simulink model "Robot_diferencial_trayectoria_senoidal"  (R2017b)
settings: Solver=VariableStepAuto  StartTime=0.0  StopTime=Tsim  MaxStep=1e-2  MinStep=1e-7  RelTol=1e-3
values from neighbouring files (symbols this model uses):
  A = 0.25    [graf.m]
  accel_limit = 15    [graf.m]
  B = 1    [graf.m]
  CI = [0 0 0]    [graf.m]
libraries: simulink_need_slupdate x1
settings Model: Creator=Raúl  LastModifiedBy=Alvaro

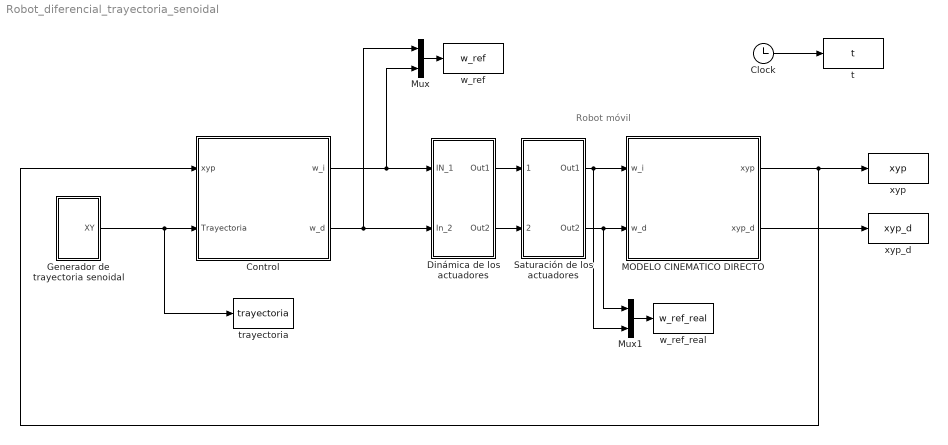
== system Robot_diferencial_trayectoria_senoidal ==
  note: Robot móvil
  Clock : Clock
  "Control " : Subsystem
  Dinámica de los actuadores : Subsystem
  Generador de trayectoria senoidal : Subsystem
  MODELO CINEMATICO DIRECTO : Subsystem
  Mux : Mux  Inputs=2
  Mux1 : Mux  Inputs=2
  Saturación de los actuadores : Subsystem
  t : ToWorkspace  VariableName=t  SampleTime=-1
  "trayectoria " : ToWorkspace  VariableName=trayectoria  SampleTime=-1
  w_ref : ToWorkspace  VariableName=w_ref  SampleTime=-1
  w_ref_real : ToWorkspace  VariableName=w_ref_real  SampleTime=-1
  xyp : ToWorkspace  VariableName=xyp  SampleTime=-1
  xyp_d : ToWorkspace  VariableName=xyp_d  SampleTime=-1
  wires:
  MODELO CINEMATICO DIRECTO/1(xyp) -> "Control "/1(xyp), xyp/1
  Clock/1 -> t/1
  Dinámica de los actuadores/1(Out1) -> Saturación de los actuadores/1(w_i_ref)
  Dinámica de los actuadores/2(Out2) -> Saturación de los actuadores/2(w_d_ref)
  "Control "/1(w_i) -> Mux/2, Dinámica de los actuadores/1(IN_1)
  "Control "/2(w_d) -> Mux/1, Dinámica de los actuadores/2(In_2)
  Mux/1 -> w_ref/1
  MODELO CINEMATICO DIRECTO/2(xyp_d) -> xyp_d/1
  Generador de trayectoria senoidal/1(XY) -> "trayectoria "/1, "Control "/2("Trayectoria ")
  Saturación de los actuadores/1(Out1) -> Mux1/2, MODELO CINEMATICO DIRECTO/1(w_i)
  Saturación de los actuadores/2(Out2) -> Mux1/1, MODELO CINEMATICO DIRECTO/2(w_d)
  Mux1/1 -> w_ref_real/1

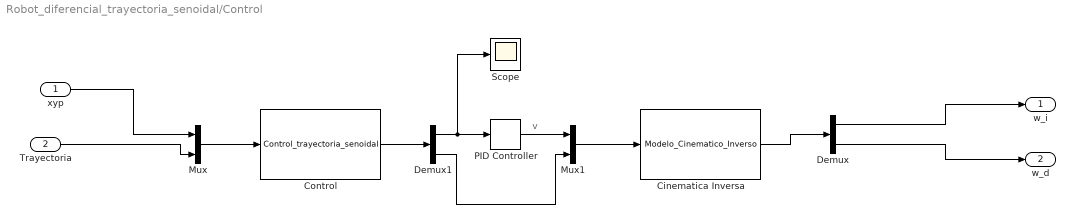
== system Robot_diferencial_trayectoria_senoidal/Control  ==
  note: v
  xyp : Inport
  "Trayectoria " : Inport  Port=2
  Cinematica Inversa : MATLABFcn  MATLABFcn=Modelo_Cinematico_Inverso  OutputDimensions=2
  "Control " : MATLABFcn  MATLABFcn=Control_trayectoria_senoidal  OutputDimensions=2
  Demux : Demux  Outputs=2
  Demux1 : Demux  Outputs=2
  Mux : Mux  Inputs=2
  Mux1 : Mux  Inputs=2
  PID Controller : simulink_need_slupdate/PID Controller  P=2.5  I=0.5  D=0
      settings: SourceProductName=Simulink
  Scope : Scope
  w_i : Outport
  w_d : Outport  Port=2
  wires:
  Demux/1 -> w_i/1
  Demux/2 -> w_d/1
  "Trayectoria "/1 -> Mux/2
  Mux/1 -> "Control "/1
  xyp/1 -> Mux/1
  Mux1/1 -> Cinematica Inversa/1
  "Control "/1 -> Demux1/1
  Demux1/1 -> Scope/1, PID Controller/1
  Demux1/2 -> Mux1/2
  PID Controller/1 -> Mux1/1
  Cinematica Inversa/1 -> Demux/1

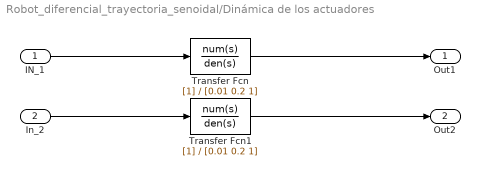
== system Robot_diferencial_trayectoria_senoidal/Dinámica de los actuadores ==
  IN_1 : Inport
  In_2 : Inport  Port=2
  Transfer Fcn : TransferFcn  Denominator=[0.01 0.2 1]
  Transfer Fcn1 : TransferFcn  Denominator=[0.01 0.2 1]
  Out1 : Outport
  Out2 : Outport  Port=2
  wires:
  Transfer Fcn1/1 -> Out2/1
  In_2/1 -> Transfer Fcn1/1
  Transfer Fcn/1 -> Out1/1
  IN_1/1 -> Transfer Fcn/1

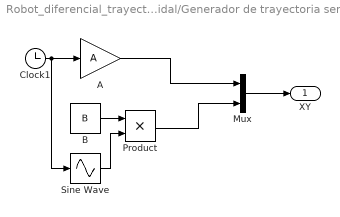
== system Robot_diferencial_trayectoria_senoidal/Generador de trayectoria senoidal ==
  A : Gain  Gain=A
  B : Constant  Value=B
  Clock1 : Clock
  Mux : Mux  Inputs=2
  Product : Product
  Sine Wave : Sin  TimeSource=Use external signal  Frequency=2*pi/10  SampleTime=0
  XY : Outport
  wires:
  Sine Wave/1 -> Product/2
  B/1 -> Product/1
  Clock1/1 -> Sine Wave/1, A/1
  Mux/1 -> XY/1
  Product/1 -> Mux/2
  A/1 -> Mux/1

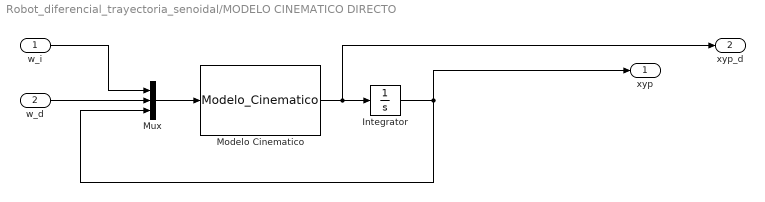
== system Robot_diferencial_trayectoria_senoidal/MODELO CINEMATICO DIRECTO ==
  w_i : Inport
  w_d : Inport  Port=2
  Integrator : Integrator  InitialCondition=CI
  "Modelo Cinematico " : MATLABFcn  MATLABFcn=Modelo_Cinematico
  Mux : Mux  Inputs=3
  xyp : Outport
  xyp_d : Outport  Port=2
  wires:
  "Modelo Cinematico "/1 -> xyp_d/1, Integrator/1
  w_i/1 -> Mux/1
  Integrator/1 -> xyp/1, Mux/3
  Mux/1 -> "Modelo Cinematico "/1
  w_d/1 -> Mux/2

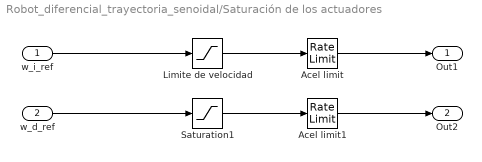
== system Robot_diferencial_trayectoria_senoidal/Saturación de los actuadores ==
  w_i_ref : Inport
  w_d_ref : Inport  Port=2
  Acel limit : RateLimiter  RisingSlewLimit=accel_limit  FallingSlewLimit=-accel_limit  SampleTimeMode=inherited
  Acel limit1 : RateLimiter  RisingSlewLimit=accel_limit  FallingSlewLimit=-accel_limit  SampleTimeMode=inherited
  Limite de velocidad : Saturate  UpperLimit=2.5  LowerLimit=-2.5
  Saturation1 : Saturate  UpperLimit=2.5  LowerLimit=-2.5
  Out1 : Outport
  Out2 : Outport  Port=2
  wires:
  w_i_ref/1 -> Limite de velocidad/1
  w_d_ref/1 -> Saturation1/1
  Limite de velocidad/1 -> Acel limit/1
  Acel limit/1 -> Out1/1
  Saturation1/1 -> Acel limit1/1
  Acel limit1/1 -> Out2/1
